simulink model "SimLab3"  (R2015b)
settings: Solver=VariableStepAuto  SolverMode=SingleTasking  StartTime=0.0  StopTime=10  RelTol=1e-3
values from neighbouring files (symbols this model uses):
  Amplitude = 20    [Lab3_1.m]    (also in Lab3_2.m; Lab3_2_discrete_disg.m)
  dm = 3.8E-6    (= 3.8e-06)    [Lab3.m]    (also in Lab3_1.m; Lab3_2.m; Lab3_2_discrete_disg.m; Lab3_3.m)
  Dpos = 0    [Lab3_1.m]    (also in Lab3_2.m; Lab3_3.m)
  Dsp = double(D)    [Lab3_1.m]    (also in Lab3_2.m; Lab3_3.m)
  Freq = 0.2    [Lab3_1.m]    (also in Lab3_2.m; Lab3_2_discrete_disg.m)
  Ipos = 0    [Lab3_1.m]    (also in Lab3_2.m; Lab3_3.m)
  Isp = double(I)    [Lab3_1.m]    (also in Lab3_2.m; Lab3_3.m)
  Jeq = Jm + (J1+J2)/(n^2)    (= 2.186e-06)    [Lab3.m]    (also in Lab3_1.m; Lab3_2.m; Lab3_2_discrete_disg.m; Lab3_3.m)
  Kemf = 1/(137*2*pi/60)    (= 0.0697028947848)    [Lab3.m]    (also in Lab3_1.m; Lab3_2.m; Lab3_2_discrete_disg.m; Lab3_3.m)
  Km = 69.7E-3    (= 0.0697)    [Lab3.m]    (also in Lab3_1.m; Lab3_2.m; Lab3_2_discrete_disg.m; Lab3_3.m)
  n = 5    [Lab3.m]    (also in Lab3_1.m; Lab3_2.m; Lab3_2_discrete_disg.m; Lab3_3.m)
  Npos = 0    [Lab3_1.m]    (also in Lab3_2.m; Lab3_3.m)
  Nsp = double(N)    [Lab3_1.m]    (also in Lab3_2.m; Lab3_3.m)
  Ppos = 1    [Lab3_1.m]    (also in Lab3_2.m; Lab3_3.m)
  Psp = double(P)    [Lab3_1.m]    (also in Lab3_2.m; Lab3_3.m)
  R = 112    [Lab3.m]    (also in Lab3_1.m; Lab3_2.m; Lab3_2_discrete_disg.m; Lab3_3.m)
  Speed_ref_step = 20    [Lab3_1.m]    (also in Lab3_2.m; Lab3_2_discrete_disg.m)
  Ts = 2E-3    (= 0.002)    [Lab3_1.m]    (also in Lab3_2.m; Lab3_2_discrete_disg.m; Lab3_4.m = 0.02; ex5LIN_param.m = 0.0005)
libraries: simulink x4
settings Model: Creator=sofianh  LastModifiedBy=diegogm
settings DataIOCC: SaveFormat=Array
settings OptimizationCC: BlockReduction=off  BooleanDataType=off
settings DebuggingCC: SaveWithParameterizedLinksMsg=none  UnderspecifiedInitializationDetection=Classic  MergeDetectMultiDrivingBlocksExec=none  SignalResolutionControl=TryResolveAllWithWarning
settings HardwareCC: ProdBitPerPointer=32  ProdLargestAtomicFloat=None  ProdIntDivRoundTo=Undefined  ProdEndianess=Unspecified  ProdWordSize=32  ProdHWDeviceType=32-bit Generic  TargetUnknown=on
settings GRTTargetCC: GeneratePreprocessorConditionals=Disable all
settings ConfigComp: CovModelRefEnable=Off  CovSFcnEnable=off

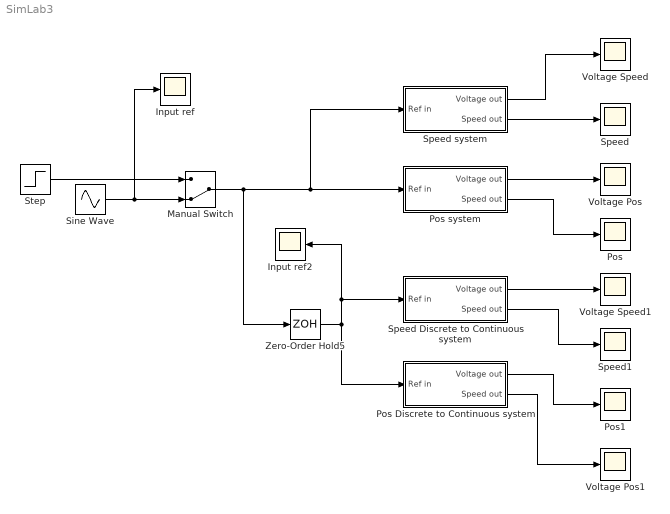
== system SimLab3 ==
  Input ref : Scope
  Input ref2 : Scope
  Manual Switch : ManualSwitch  CurrentSetting=0
  Pos : Scope
  Pos Discrete to Continuous system : Subsystem
  "Pos system " : Subsystem
  Pos1 : Scope
  Sine Wave : Sin  Amplitude=Amplitude  Frequency=Freq*10  SampleTime=0
  Speed : Scope
  Speed Discrete to Continuous system : Subsystem
  Speed system : Subsystem
  Speed1 : Scope
  Step : Step  Time=0  After=Speed_ref_step  SampleTime=0
  Voltage Pos : Scope
  Voltage Pos1 : Scope
  Voltage Speed : Scope
  Voltage Speed1 : Scope
  Zero-Order Hold5 : ZeroOrderHold  SampleTime=Ts
  wires:
  Step/1 -> Manual Switch/1
  Sine Wave/1 -> Input ref/1, Manual Switch/2
  Speed system/1(Voltage out) -> Voltage Speed/1
  Speed system/2(Speed out) -> Speed/1
  "Pos system "/2(Speed out) -> Pos/1
  "Pos system "/1(Voltage out) -> Voltage Pos/1
  Manual Switch/1 -> Zero-Order Hold5/1, "Pos system "/1(Ref in), Speed system/1(Ref in)
  Zero-Order Hold5/1 -> Speed Discrete to Continuous system/1(Ref in), Input ref2/1, Pos Discrete to Continuous system/1(Ref in)
  Speed Discrete to Continuous system/1(Voltage out) -> Voltage Speed1/1
  Speed Discrete to Continuous system/2(Speed out) -> Speed1/1
  Pos Discrete to Continuous system/1(Voltage out) -> Pos1/1
  Pos Discrete to Continuous system/2(Speed out) -> Voltage Pos1/1

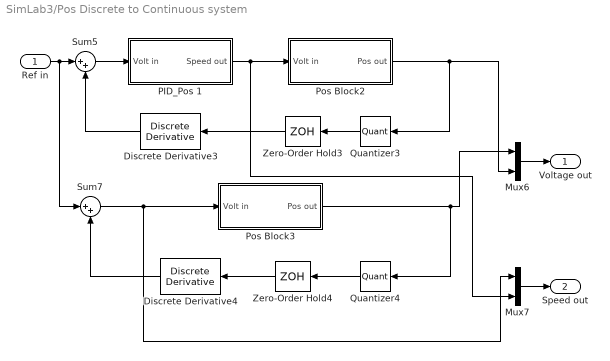
== system SimLab3/Pos Discrete to Continuous system ==
  Ref in : Inport
  Discrete Derivative3 : simulink/Discrete/Discrete Derivative  gainval=1.0  ICPrevScaledInput=0.0  InputProcessing=Inherited  OutMin=[]  OutMax=[]  OutDataType=fixdt(1, 16)  OutScaling=2^-10  DoSatur=off
  Discrete Derivative4 : simulink/Discrete/Discrete Derivative  gainval=1.0  ICPrevScaledInput=0.0  InputProcessing=Inherited  OutMin=[]  OutMax=[]  OutDataType=fixdt(1, 16)  OutScaling=2^-10  DoSatur=off
  Mux6 : Mux  Inputs=2
  Mux7 : Mux  Inputs=2
  PID_Pos 1 : Subsystem
  Pos Block2 : Subsystem
  Pos Block3 : Subsystem
  Quantizer3 : Quantizer  QuantizationInterval=Pulses  LinearizeAsGain=off  SampleTime=Ts
  Quantizer4 : Quantizer  QuantizationInterval=Pulses  LinearizeAsGain=off  SampleTime=Ts
  Sum5 : Sum  Inputs=|++
  Sum7 : Sum  Inputs=|++
  Zero-Order Hold3 : ZeroOrderHold  SampleTime=Ts
  Zero-Order Hold4 : ZeroOrderHold  SampleTime=Ts
  Voltage out : Outport
  Speed out : Outport  Port=2
  wires:
  Sum5/1 -> PID_Pos 1/1(Volt in)
  PID_Pos 1/1(Speed out) -> Pos Block2/1(Volt in), Mux7/2
  Mux6/1 -> Voltage out/1
  Sum7/1 -> Mux7/1, Pos Block3/1(Volt in)
  Mux7/1 -> Speed out/1
  Pos Block2/1("Pos out ") -> Quantizer3/1, Mux6/2
  Quantizer3/1 -> Zero-Order Hold3/1
  Zero-Order Hold3/1 -> Discrete Derivative3/1
  Discrete Derivative3/1 -> Sum5/2
  Pos Block3/1("Pos out ") -> Quantizer4/1, Mux6/1
  Quantizer4/1 -> Zero-Order Hold4/1
  Zero-Order Hold4/1 -> Discrete Derivative4/1
  Discrete Derivative4/1 -> Sum7/2
  Ref in/1 -> Sum7/1, Sum5/1

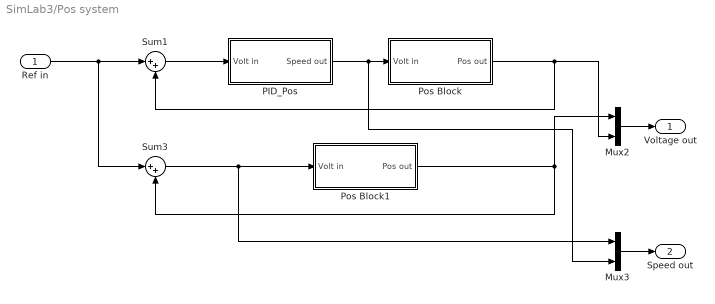
== system SimLab3/Pos system  ==
  Ref in : Inport
  Mux2 : Mux  Inputs=2
  Mux3 : Mux  Inputs=2
  "PID_Pos " : Subsystem
  Pos Block : Subsystem
  Pos Block1 : Subsystem
  Sum1 : Sum  Inputs=|++
  Sum3 : Sum  Inputs=|++
  Voltage out : Outport
  Speed out : Outport  Port=2
  wires:
  Ref in/1 -> Sum1/1, Sum3/1
  Sum1/1 -> "PID_Pos "/1(Volt in)
  "PID_Pos "/1(Speed out) -> Mux3/2, Pos Block/1(Volt in)
  Pos Block1/1("Pos out ") -> Sum3/2, Mux2/1
  Mux2/1 -> Voltage out/1
  Pos Block/1("Pos out ") -> Sum1/2, Mux2/2
  Sum3/1 -> Mux3/1, Pos Block1/1(Volt in)
  Mux3/1 -> Speed out/1

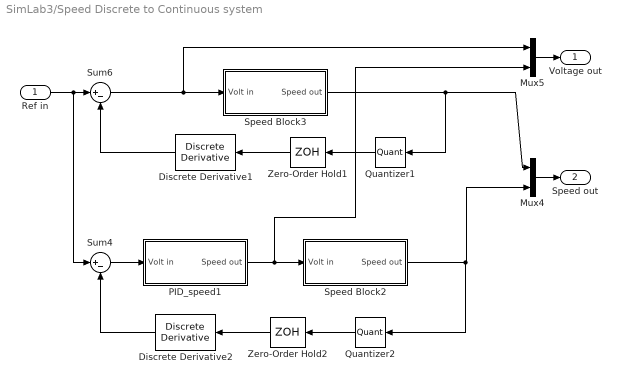
== system SimLab3/Speed Discrete to Continuous system ==
  Ref in : Inport
  Discrete Derivative1 : simulink/Discrete/Discrete Derivative  gainval=1.0  ICPrevScaledInput=0.0  InputProcessing=Inherited  OutMin=[]  OutMax=[]  OutDataType=fixdt(1, 16)  OutScaling=2^-10  DoSatur=off
  Discrete Derivative2 : simulink/Discrete/Discrete Derivative  gainval=1.0  ICPrevScaledInput=0.0  InputProcessing=Inherited  OutMin=[]  OutMax=[]  OutDataType=fixdt(1, 16)  OutScaling=2^-10  DoSatur=off
  Mux4 : Mux  Inputs=2
  Mux5 : Mux  Inputs=2
  PID_speed1 : Subsystem
  Quantizer1 : Quantizer  QuantizationInterval=Pulses  LinearizeAsGain=off  SampleTime=Ts
  Quantizer2 : Quantizer  QuantizationInterval=Pulses  LinearizeAsGain=off  SampleTime=Ts
  Speed Block2 : Subsystem
  Speed Block3 : Subsystem
  Sum4 : Sum  Inputs=|+-
  Sum6 : Sum  Inputs=|+-
  Zero-Order Hold1 : ZeroOrderHold  SampleTime=Ts
  Zero-Order Hold2 : ZeroOrderHold  SampleTime=Ts
  Voltage out : Outport
  Speed out : Outport  Port=2
  wires:
  Ref in/1 -> Sum4/1, Sum6/1
  Sum4/1 -> PID_speed1/1(Volt in)
  PID_speed1/1(Speed out) -> Mux5/2, Speed Block2/1(Volt in)
  Speed Block3/1(Speed out) -> Quantizer1/1, Mux4/1
  Sum6/1 -> Mux5/1, Speed Block3/1(Volt in)
  Mux4/1 -> Speed out/1
  Mux5/1 -> Voltage out/1
  Quantizer1/1 -> Zero-Order Hold1/1
  Zero-Order Hold1/1 -> Discrete Derivative1/1
  Discrete Derivative1/1 -> Sum6/2
  Speed Block2/1(Speed out) -> Quantizer2/1, Mux4/2
  Quantizer2/1 -> Zero-Order Hold2/1
  Zero-Order Hold2/1 -> Discrete Derivative2/1
  Discrete Derivative2/1 -> Sum4/2

== system SimLab3/Speed system ==
  Ref in : Inport
  Mux : Mux  Inputs=2
  Mux1 : Mux  Inputs=2
  PID_speed : Subsystem
  Speed Block : Subsystem
  Speed Block1 : Subsystem
  Sum : Sum  Inputs=|+-
  Sum2 : Sum  Inputs=|+-
  Voltage out : Outport
  Speed out : Outport  Port=2
  wires:
  Speed Block/1(Speed out) -> Sum/2, Mux/2
  Sum/1 -> PID_speed/1(Volt in)
  PID_speed/1(Speed out) -> Mux1/2, Speed Block/1(Volt in)
  Speed Block1/1(Speed out) -> Sum2/2, Mux/1
  Sum2/1 -> Mux1/1, Speed Block1/1(Volt in)
  Mux/1 -> Speed out/1
  Mux1/1 -> Voltage out/1
  Ref in/1 -> Sum/1, Sum2/1

== system SimLab3/Pos Discrete to Continuous system/PID_Pos 1 ==
  Volt in : Inport
  Derivative Gain : Gain  Gain=Dpos
  Filter Gain : Gain  Gain=Npos
  Integral Gain : Gain  Gain=Ipos
  Integrator : Integrator
  Integrator1 : Integrator
  Proportional Gain : Gain  Gain=Ppos
  Sum : Sum  Inputs=|+-
  Sum1 : Sum  Inputs=+++
  Speed out : Outport
  wires:
  Sum1/1 -> Speed out/1
  Integrator/1 -> Sum1/2
  Integrator1/1 -> Sum/2
  Filter Gain/1 -> Sum1/3, Integrator1/1
  Sum/1 -> Filter Gain/1
  Derivative Gain/1 -> Sum/1
  Integral Gain/1 -> Integrator/1
  Proportional Gain/1 -> Sum1/1
  Volt in/1 -> Derivative Gain/1, Integral Gain/1, Proportional Gain/1

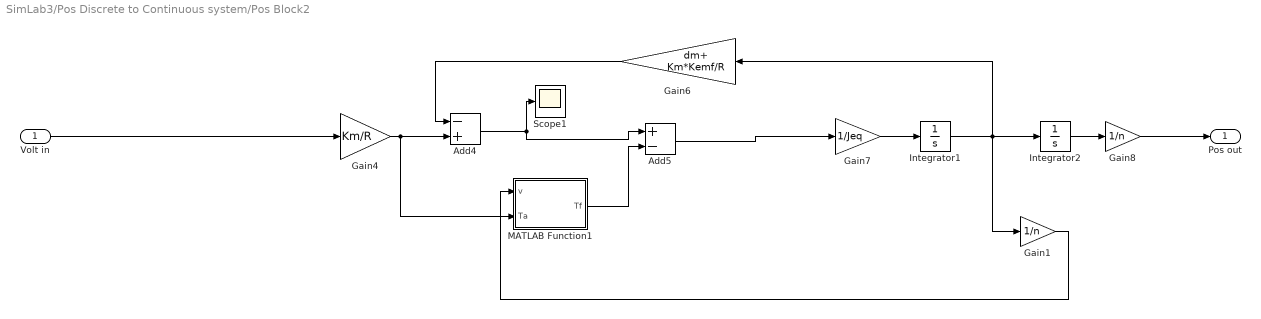
== system SimLab3/Pos Discrete to Continuous system/Pos Block2 ==
  Volt in : Inport
  Add4 : Sum  Inputs=-+
  Add5 : Sum  Inputs=+-
  Gain1 : Gain  Gain=1/n
  Gain4 : Gain  Gain=Km/R
  Gain6 : Gain  Gain=dm+ Km*Kemf/R
  Gain7 : Gain  Gain=1/Jeq
  Gain8 : Gain  Gain=1/n
  Integrator1 : Integrator
  Integrator2 : Integrator
  MATLAB Function1 : MATLAB Function  TreatAsAtomicUnit=on
  Scope1 : Scope
  "Pos out " : Outport
  wires:
  Gain4/1 -> MATLAB Function1/2(Ta), Add4/2
  Integrator1/1 -> Integrator2/1, Gain1/1, Gain6/1
  Gain6/1 -> Add4/1
  Gain7/1 -> Integrator1/1
  Integrator2/1 -> Gain8/1
  Gain1/1 -> MATLAB Function1/1(v)
  Volt in/1 -> Gain4/1
  Add5/1 -> Gain7/1
  Add4/1 -> Add5/1, Scope1/1
  MATLAB Function1/1(Tf) -> Add5/2
  Gain8/1 -> "Pos out "/1

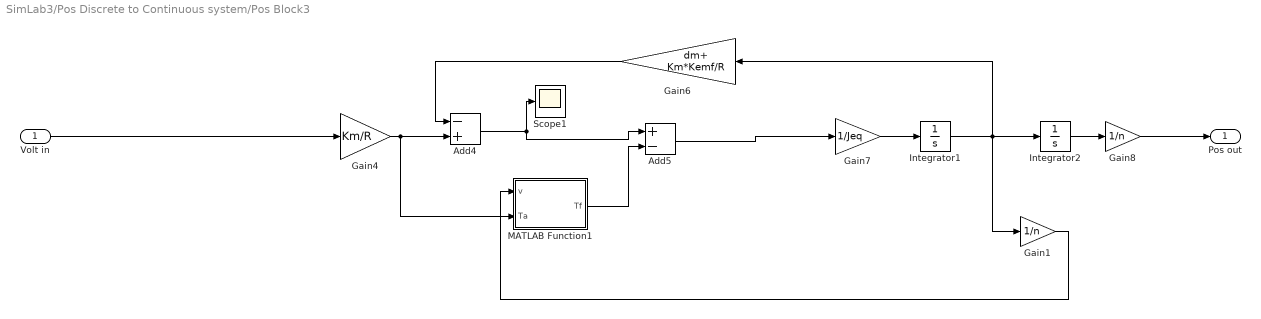
== system SimLab3/Pos Discrete to Continuous system/Pos Block3 ==
  Volt in : Inport
  Add4 : Sum  Inputs=-+
  Add5 : Sum  Inputs=+-
  Gain1 : Gain  Gain=1/n
  Gain4 : Gain  Gain=Km/R
  Gain6 : Gain  Gain=dm+ Km*Kemf/R
  Gain7 : Gain  Gain=1/Jeq
  Gain8 : Gain  Gain=1/n
  Integrator1 : Integrator
  Integrator2 : Integrator
  MATLAB Function1 : MATLAB Function  TreatAsAtomicUnit=on
  Scope1 : Scope
  "Pos out " : Outport
  wires:
  Gain4/1 -> MATLAB Function1/2(Ta), Add4/2
  Integrator1/1 -> Integrator2/1, Gain1/1, Gain6/1
  Gain6/1 -> Add4/1
  Gain7/1 -> Integrator1/1
  Integrator2/1 -> Gain8/1
  Gain1/1 -> MATLAB Function1/1(v)
  Volt in/1 -> Gain4/1
  Add5/1 -> Gain7/1
  Add4/1 -> Add5/1, Scope1/1
  MATLAB Function1/1(Tf) -> Add5/2
  Gain8/1 -> "Pos out "/1

== system SimLab3/Pos system /PID_Pos  ==
  Volt in : Inport
  Derivative Gain : Gain  Gain=Dpos
  Filter Gain : Gain  Gain=Npos
  Integral Gain : Gain  Gain=Ipos
  Integrator : Integrator
  Integrator1 : Integrator
  Proportional Gain : Gain  Gain=Ppos
  Sum : Sum  Inputs=|+-
  Sum1 : Sum  Inputs=+++
  Speed out : Outport
  wires:
  Sum1/1 -> Speed out/1
  Integrator/1 -> Sum1/2
  Integrator1/1 -> Sum/2
  Filter Gain/1 -> Sum1/3, Integrator1/1
  Sum/1 -> Filter Gain/1
  Derivative Gain/1 -> Sum/1
  Integral Gain/1 -> Integrator/1
  Proportional Gain/1 -> Sum1/1
  Volt in/1 -> Derivative Gain/1, Integral Gain/1, Proportional Gain/1

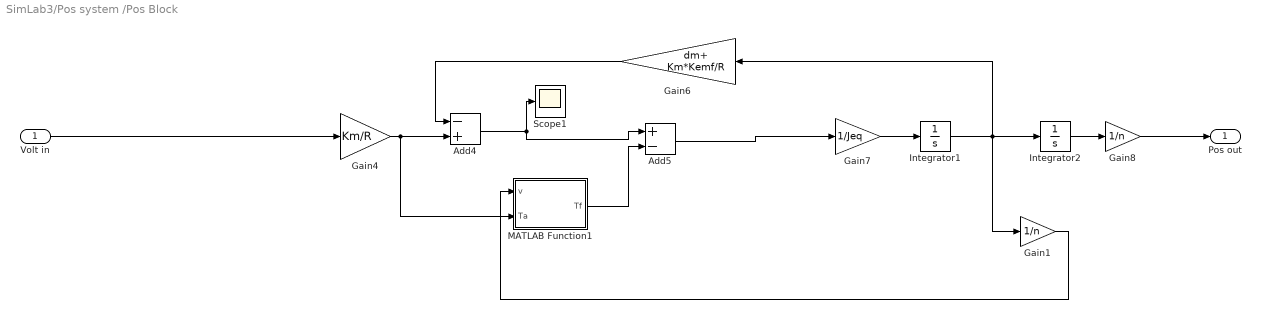
== system SimLab3/Pos system /Pos Block ==
  Volt in : Inport
  Add4 : Sum  Inputs=-+
  Add5 : Sum  Inputs=+-
  Gain1 : Gain  Gain=1/n
  Gain4 : Gain  Gain=Km/R
  Gain6 : Gain  Gain=dm+ Km*Kemf/R
  Gain7 : Gain  Gain=1/Jeq
  Gain8 : Gain  Gain=1/n
  Integrator1 : Integrator
  Integrator2 : Integrator
  MATLAB Function1 : MATLAB Function  TreatAsAtomicUnit=on
  Scope1 : Scope
  "Pos out " : Outport
  wires:
  Gain4/1 -> MATLAB Function1/2(Ta), Add4/2
  Integrator1/1 -> Integrator2/1, Gain1/1, Gain6/1
  Gain6/1 -> Add4/1
  Gain7/1 -> Integrator1/1
  Integrator2/1 -> Gain8/1
  Gain1/1 -> MATLAB Function1/1(v)
  Volt in/1 -> Gain4/1
  Add5/1 -> Gain7/1
  Add4/1 -> Add5/1, Scope1/1
  MATLAB Function1/1(Tf) -> Add5/2
  Gain8/1 -> "Pos out "/1

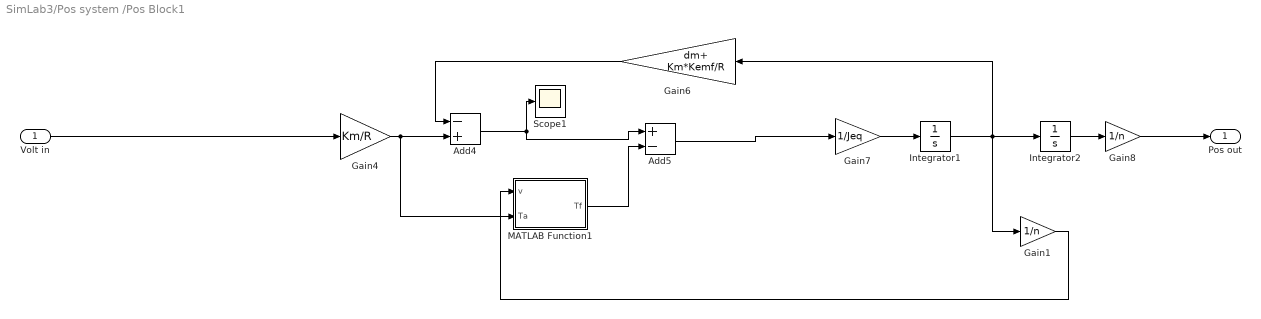
== system SimLab3/Pos system /Pos Block1 ==
  Volt in : Inport
  Add4 : Sum  Inputs=-+
  Add5 : Sum  Inputs=+-
  Gain1 : Gain  Gain=1/n
  Gain4 : Gain  Gain=Km/R
  Gain6 : Gain  Gain=dm+ Km*Kemf/R
  Gain7 : Gain  Gain=1/Jeq
  Gain8 : Gain  Gain=1/n
  Integrator1 : Integrator
  Integrator2 : Integrator
  MATLAB Function1 : MATLAB Function  TreatAsAtomicUnit=on
  Scope1 : Scope
  "Pos out " : Outport
  wires:
  Gain4/1 -> MATLAB Function1/2(Ta), Add4/2
  Integrator1/1 -> Integrator2/1, Gain1/1, Gain6/1
  Gain6/1 -> Add4/1
  Gain7/1 -> Integrator1/1
  Integrator2/1 -> Gain8/1
  Gain1/1 -> MATLAB Function1/1(v)
  Volt in/1 -> Gain4/1
  Add5/1 -> Gain7/1
  Add4/1 -> Add5/1, Scope1/1
  MATLAB Function1/1(Tf) -> Add5/2
  Gain8/1 -> "Pos out "/1

== system SimLab3/Speed Discrete to Continuous system/PID_speed1 ==
  Volt in : Inport
  Derivative Gain : Gain  Gain=Dsp
  Filter Gain : Gain  Gain=Nsp
  Integral Gain : Gain  Gain=Isp
  Integrator : Integrator
  Integrator1 : Integrator
  Proportional Gain : Gain  Gain=Psp
  Sum : Sum  Inputs=|+-
  Sum1 : Sum  Inputs=+++
  Speed out : Outport
  wires:
  Sum1/1 -> Speed out/1
  Integrator/1 -> Sum1/2
  Integrator1/1 -> Sum/2
  Filter Gain/1 -> Sum1/3, Integrator1/1
  Sum/1 -> Filter Gain/1
  Derivative Gain/1 -> Sum/1
  Integral Gain/1 -> Integrator/1
  Proportional Gain/1 -> Sum1/1
  Volt in/1 -> Derivative Gain/1, Integral Gain/1, Proportional Gain/1

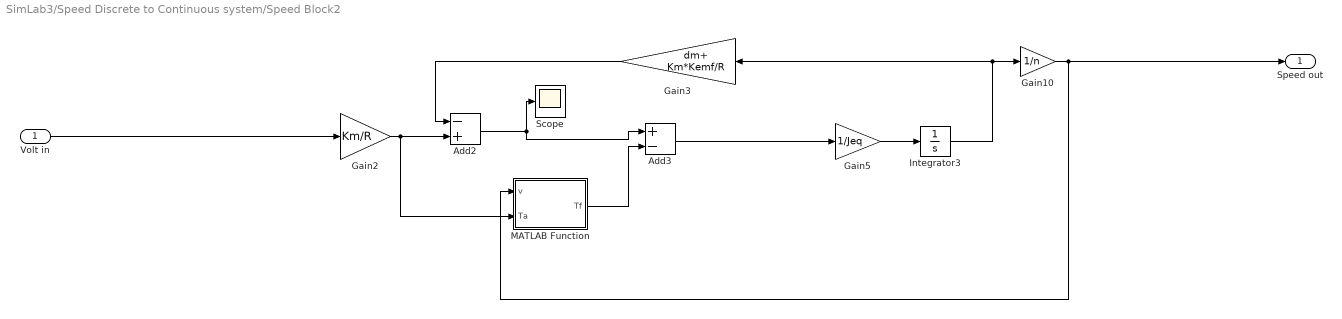
== system SimLab3/Speed Discrete to Continuous system/Speed Block2 ==
  Volt in : Inport
  Add2 : Sum  Inputs=-+
  Add3 : Sum  Inputs=+-
  Gain10 : Gain  Gain=1/n
  Gain2 : Gain  Gain=Km/R
  Gain3 : Gain  Gain=dm+ Km*Kemf/R
  Gain5 : Gain  Gain=1/Jeq
  Integrator3 : Integrator
  MATLAB Function : MATLAB Function  TreatAsAtomicUnit=on
  Scope : Scope
  Speed out : Outport
  wires:
  Gain2/1 -> MATLAB Function/2(Ta), Add2/2
  Integrator3/1 -> Gain10/1, Gain3/1
  Gain3/1 -> Add2/1
  Gain5/1 -> Integrator3/1
  Gain10/1 -> Speed out/1, MATLAB Function/1(v)
  Volt in/1 -> Gain2/1
  Add3/1 -> Gain5/1
  Add2/1 -> Add3/1, Scope/1
  MATLAB Function/1(Tf) -> Add3/2

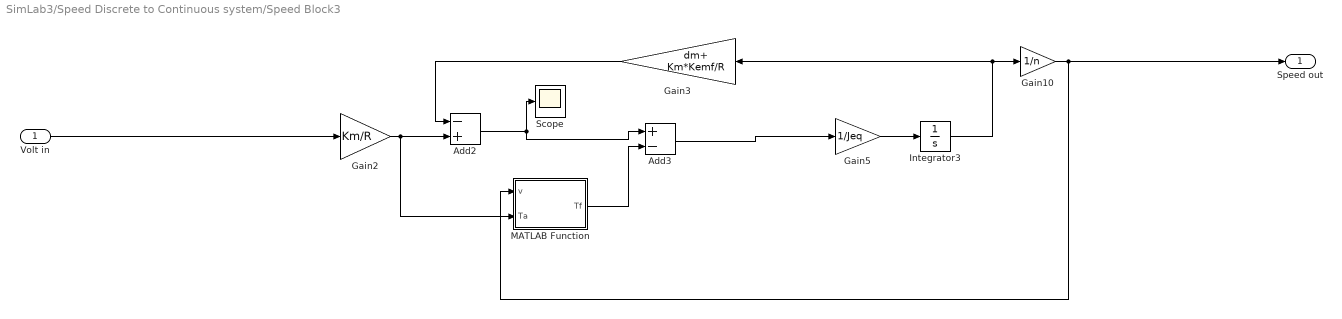
== system SimLab3/Speed Discrete to Continuous system/Speed Block3 ==
  Volt in : Inport
  Add2 : Sum  Inputs=-+
  Add3 : Sum  Inputs=+-
  Gain10 : Gain  Gain=1/n
  Gain2 : Gain  Gain=Km/R
  Gain3 : Gain  Gain=dm+ Km*Kemf/R
  Gain5 : Gain  Gain=1/Jeq
  Integrator3 : Integrator
  MATLAB Function : MATLAB Function  TreatAsAtomicUnit=on
  Scope : Scope
  Speed out : Outport
  wires:
  Gain2/1 -> MATLAB Function/2(Ta), Add2/2
  Integrator3/1 -> Gain10/1, Gain3/1
  Gain3/1 -> Add2/1
  Gain5/1 -> Integrator3/1
  Gain10/1 -> Speed out/1, MATLAB Function/1(v)
  Volt in/1 -> Gain2/1
  Add3/1 -> Gain5/1
  Add2/1 -> Add3/1, Scope/1
  MATLAB Function/1(Tf) -> Add3/2

== system SimLab3/Speed system/PID_speed ==
  Volt in : Inport
  Derivative Gain : Gain  Gain=Dsp
  Filter Gain : Gain  Gain=Nsp
  Integral Gain : Gain  Gain=Isp
  Integrator : Integrator
  Integrator1 : Integrator
  Proportional Gain : Gain  Gain=Psp
  Sum : Sum  Inputs=|+-
  Sum1 : Sum  Inputs=+++
  Speed out : Outport
  wires:
  Sum1/1 -> Speed out/1
  Integrator/1 -> Sum1/2
  Integrator1/1 -> Sum/2
  Filter Gain/1 -> Sum1/3, Integrator1/1
  Sum/1 -> Filter Gain/1
  Derivative Gain/1 -> Sum/1
  Integral Gain/1 -> Integrator/1
  Proportional Gain/1 -> Sum1/1
  Volt in/1 -> Derivative Gain/1, Integral Gain/1, Proportional Gain/1

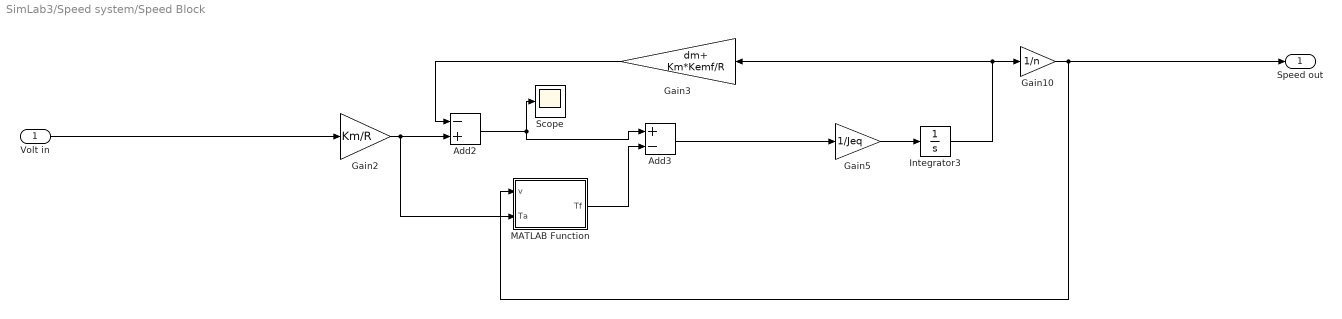
== system SimLab3/Speed system/Speed Block ==
  Volt in : Inport
  Add2 : Sum  Inputs=-+
  Add3 : Sum  Inputs=+-
  Gain10 : Gain  Gain=1/n
  Gain2 : Gain  Gain=Km/R
  Gain3 : Gain  Gain=dm+ Km*Kemf/R
  Gain5 : Gain  Gain=1/Jeq
  Integrator3 : Integrator
  MATLAB Function : MATLAB Function  TreatAsAtomicUnit=on
  Scope : Scope
  Speed out : Outport
  wires:
  Gain2/1 -> MATLAB Function/2(Ta), Add2/2
  Integrator3/1 -> Gain10/1, Gain3/1
  Gain3/1 -> Add2/1
  Gain5/1 -> Integrator3/1
  Gain10/1 -> Speed out/1, MATLAB Function/1(v)
  Volt in/1 -> Gain2/1
  Add3/1 -> Gain5/1
  Add2/1 -> Add3/1, Scope/1
  MATLAB Function/1(Tf) -> Add3/2

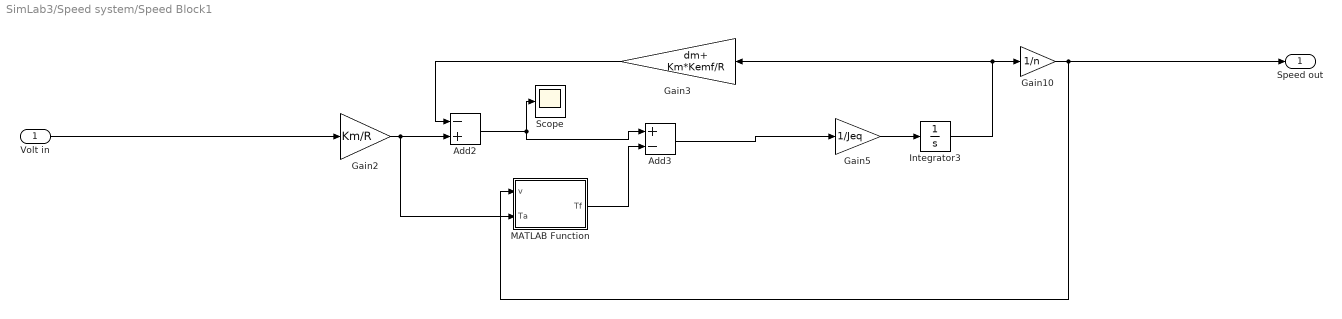
== system SimLab3/Speed system/Speed Block1 ==
  Volt in : Inport
  Add2 : Sum  Inputs=-+
  Add3 : Sum  Inputs=+-
  Gain10 : Gain  Gain=1/n
  Gain2 : Gain  Gain=Km/R
  Gain3 : Gain  Gain=dm+ Km*Kemf/R
  Gain5 : Gain  Gain=1/Jeq
  Integrator3 : Integrator
  MATLAB Function : MATLAB Function  TreatAsAtomicUnit=on
  Scope : Scope
  Speed out : Outport
  wires:
  Gain2/1 -> MATLAB Function/2(Ta), Add2/2
  Integrator3/1 -> Gain10/1, Gain3/1
  Gain3/1 -> Add2/1
  Gain5/1 -> Integrator3/1
  Gain10/1 -> Speed out/1, MATLAB Function/1(v)
  Volt in/1 -> Gain2/1
  Add3/1 -> Gain5/1
  Add2/1 -> Add3/1, Scope/1
  MATLAB Function/1(Tf) -> Add3/2

== matlab function SimLab3/Pos system /Pos Block/MATLAB Function1 ==
  data: v input; Tf output; Ta input
function Tf = fcn(v,Ta)
Tc = 1e-3;
dv = 1e-1;
if abs(v) < dv
    if abs(Ta) > Tc
        Tf = Tc*sign(Ta);
    else
        Tf = Ta;
    end
else
    Tf = Tc*sign(v);
end

== matlab function SimLab3/Speed system/Speed Block1/MATLAB Function ==
  data: v input; Tf output; Ta input
function Tf = fcn(v,Ta)
Tc = 1e-3;
dv = 1e-1;
if abs(v) < dv
    if abs(Ta) > Tc
        Tf = Tc*sign(Ta);
    else
        Tf = Ta;
    end
else
    Tf = Tc*sign(v);
end

== matlab function SimLab3/Speed system/Speed Block/MATLAB Function ==
  data: v input; Tf output; Ta input
function Tf = fcn(v,Ta)
Tc = 1e-3;
dv = 1e-1;
if abs(v) < dv
    if abs(Ta) > Tc
        Tf = Tc*sign(Ta);
    else
        Tf = Ta;
    end
else
    Tf = Tc*sign(v);
end

== matlab function SimLab3/Pos system /Pos Block1/MATLAB Function1 ==
  data: v input; Tf output; Ta input
function Tf = fcn(v,Ta)
Tc = 1e-3;
dv = 1e-1;
if abs(v) < dv
    if abs(Ta) > Tc
        Tf = Tc*sign(Ta);
    else
        Tf = Ta;
    end
else
    Tf = Tc*sign(v);
end

== matlab function SimLab3/Pos Discrete to Continuous system/Pos Block2/MATLAB Function1 ==
  data: v input; Tf output; Ta input
function Tf = fcn(v,Ta)
Tc = 1e-3;
dv = 1e-1;
if abs(v) < dv
    if abs(Ta) > Tc
        Tf = Tc*sign(Ta);
    else
        Tf = Ta;
    end
else
    Tf = Tc*sign(v);
end

== matlab function SimLab3/Pos Discrete to Continuous system/Pos Block3/MATLAB Function1 ==
  data: v input; Tf output; Ta input
function Tf = fcn(v,Ta)
Tc = 1e-3;
dv = 1e-1;
if abs(v) < dv
    if abs(Ta) > Tc
        Tf = Tc*sign(Ta);
    else
        Tf = Ta;
    end
else
    Tf = Tc*sign(v);
end

== matlab function SimLab3/Speed Discrete to Continuous system/Speed Block2/MATLAB Function ==
  data: v input; Tf output; Ta input
function Tf = fcn(v,Ta)
Tc = 1e-3;
dv = 1e-1;
if abs(v) < dv
    if abs(Ta) > Tc
        Tf = Tc*sign(Ta);
    else
        Tf = Ta;
    end
else
    Tf = Tc*sign(v);
end

== matlab function SimLab3/Speed Discrete to Continuous system/Speed Block3/MATLAB Function ==
  data: v input; Tf output; Ta input
function Tf = fcn(v,Ta)
Tc = 1e-3;
dv = 1e-1;
if abs(v) < dv
    if abs(Ta) > Tc
        Tf = Tc*sign(Ta);
    else
        Tf = Ta;
    end
else
    Tf = Tc*sign(v);
end
